simulink model "mySimpleODEwithInp1"  (R2017b)
settings: Solver=ode45  StartTime=0.0  StopTime=10.0  MaxStep=0.1  RelTol=1e-3  EnableMultiTasking=on
settings Model: Creator=gfaineko  LastModifiedBy=apelttom
settings DataIOCC: SaveFormat=Array  SaveState=on  DSMLogging=off
settings OptimizationCC: LifeSpan=inf
settings DebuggingCC: UnderspecifiedInitializationDetection=Classic  MergeDetectMultiDrivingBlocksExec=none  SolverPrmCheckMsg=warning  StateNameClashWarn=warning  SFUnexpectedBacktrackingDiag=warning  SFNoUnconditionalDefaultTransitionDiag=warning  SFExecutionAtInitializationDiag=none
settings HardwareCC: ProdBitPerPointer=32  ProdBitPerSizeT=32  ProdBitPerPtrDiffT=32  ProdLargestAtomicFloat=None  ProdIntDivRoundTo=Undefined  ProdEndianess=Unspecified  ProdWordSize=32  ProdHWDeviceType=32-bit Generic
settings ModelReferenceCC: PropagateSignalLabelsOutOfModel=off
settings CodeAppCC: StateflowObjectComments=on
settings GRTTargetCC: TargetLangStandard=C89/C90 (ANSI)  GeneratePreprocessorConditionals=Disable all
settings ConfigComp: CovMetricSettings=dw  CovHtmlReporting=on  CovSaveCumulativeToWorkspaceVar=on  CovSaveSingleToWorkspaceVar=on  CovExternalEMLEnable=off

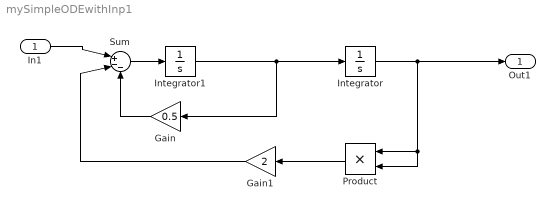
== system mySimpleODEwithInp1 ==
  In1 : Inport
  Gain : Gain  Gain=0.5
  Gain1 : Gain  Gain=2
  Integrator : Integrator
  Integrator1 : Integrator
  Product : Product
  Sum : Sum  Inputs=|+--
  Out1 : Outport
  wires:
  Integrator/1 -> Product/2, Product/1, Out1/1
  In1/1 -> Sum/1
  Sum/1 -> Integrator1/1
  Gain1/1 -> Sum/2
  Gain/1 -> Sum/3
  Integrator1/1 -> Gain/1, Integrator/1
  Product/1 -> Gain1/1
